simulink model "CPM"  (R2021a)
settings: Solver=VariableStepAuto  StartTime=0.0  StopTime=10.0  RelTol=1e-3
undefined symbols (not defined in the file or in its folder): robot
libraries: robotmaniplib x11, robotcorelib x2, dspinverses x1
settings Model: Creator=ajosh  LastModifiedBy=mluser
settings SolverCC: AlgebraicLoopSolver=TrustRegion
settings OptimizationCC: BlockReduction=off  DefaultParameterBehavior=Inlined  BufferReuse=off
settings DebuggingCC: SFMachineParentedDataDiag=warning

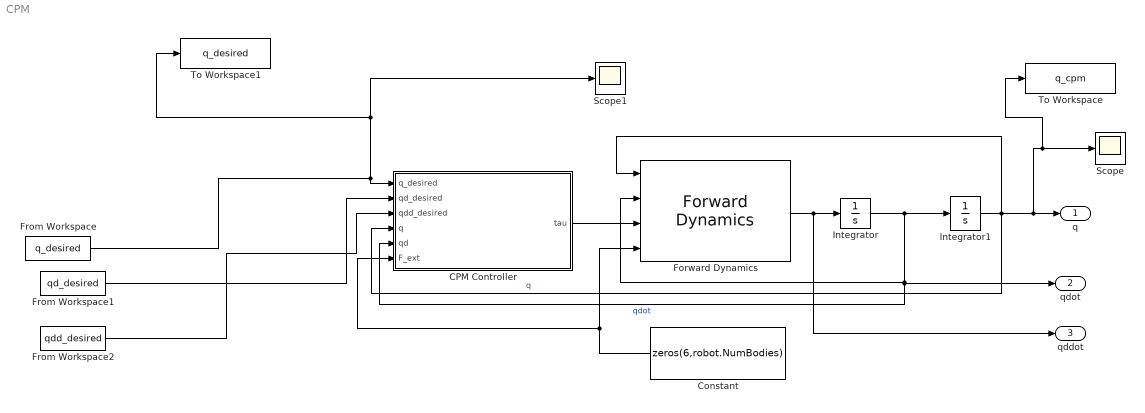
== system CPM ==
  "CPM Controller " : Subsystem
  Constant : Constant  Value=zeros(6,robot.NumBodies)
  Forward Dynamics : robotmaniplib/Forward Dynamics  RigidBodyTree=robot  SimulateUsing=Interpreted execution
  From Workspace : FromWorkspace  VariableName=q_desired  SampleTime=-1
  From Workspace1 : FromWorkspace  VariableName=qd_desired  SampleTime=-1
  From Workspace2 : FromWorkspace  VariableName=qdd_desired  SampleTime=-1
  Integrator : Integrator
  Integrator1 : Integrator
  Scope : Scope
  Scope1 : Scope
  To Workspace : ToWorkspace  VariableName=q_cpm  SaveFormat=Timeseries  SampleTime=-1
  To Workspace1 : ToWorkspace  VariableName=q_desired  SaveFormat=Timeseries  SampleTime=-1
  q : Outport
  qdot : Outport  Port=2
  qddot : Outport  Port=3
  wires:
  Forward Dynamics/1 -> Integrator/1, qddot/1
  Integrator/1 -> Integrator1/1, "CPM Controller "/5(qd), qdot/1, Forward Dynamics/2  "qdot"
  "CPM Controller "/1(tau) -> Forward Dynamics/3
  Integrator1/1 -> Forward Dynamics/1, To Workspace/1, Scope/1, q/1, "CPM Controller "/4(q)  "q"
  Constant/1 -> "CPM Controller "/6(F_ext), Forward Dynamics/4
  From Workspace/1 -> Scope1/1, To Workspace1/1, "CPM Controller "/1(q_desired)
  From Workspace1/1 -> "CPM Controller "/2(qd_desired)
  From Workspace2/1 -> "CPM Controller "/3(qdd_desired)

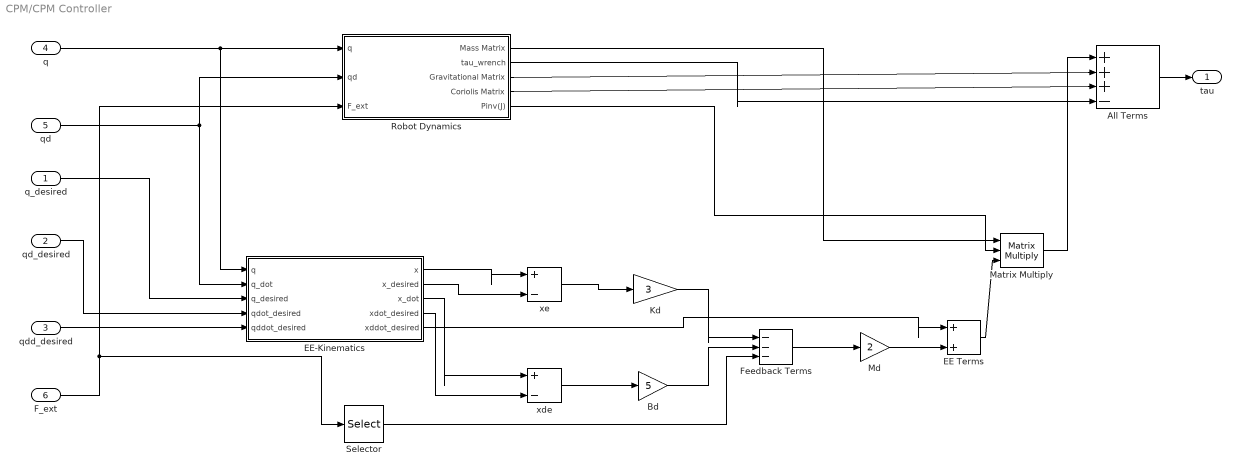
== system CPM/CPM Controller  ==
  q_desired : Inport
  qd_desired : Inport  Port=2
  qdd_desired : Inport  Port=3
  q : Inport  Port=4
  qd : Inport  Port=5
  F_ext : Inport  Port=6
  All Terms : Sum  Inputs=|+++-
  Bd : Gain  Gain=5
  EE Terms : Sum  Inputs=|++
  EE-Kinematics : Subsystem
  Feedback Terms : Sum  Inputs=|---
  Kd : Gain  Gain=3
  Matrix Multiply : Product  Inputs=3  Multiplication=Matrix(*)
  Md : Gain  Gain=2
  Robot Dynamics : Subsystem
  Selector : Selector  NumberOfDimensions=2  InputPortWidth=3  IndexOptions=Index vector (dialog),Index vector (dialog)  Indices=[1 2 3 4 5 6],2  OutputSizes=1,1
  xde : Sum  Inputs=|+-
  xe : Sum  Inputs=|+-
  tau : Outport
  wires:
  qd/1 -> EE-Kinematics/2(q_dot), Robot Dynamics/2(qd)
  xe/1 -> Kd/1
  xde/1 -> Bd/1
  Kd/1 -> Feedback Terms/1
  Bd/1 -> Feedback Terms/2
  q_desired/1 -> EE-Kinematics/3(q_desired)
  qd_desired/1 -> EE-Kinematics/4(qdot_desired)
  qdd_desired/1 -> EE-Kinematics/5(qddot_desired)
  q/1 -> EE-Kinematics/1(q), Robot Dynamics/1(q)
  EE-Kinematics/1(x) -> xe/1
  EE-Kinematics/2(x_desired) -> xe/2
  EE-Kinematics/3(x_dot) -> xde/1
  EE-Kinematics/4(xdot_desired) -> xde/2
  F_ext/1 -> Selector/1, Robot Dynamics/3(F_ext)
  Feedback Terms/1 -> Md/1
  Md/1 -> EE Terms/2
  EE-Kinematics/5(xddot_desired) -> EE Terms/1
  Robot Dynamics/1(Mass Matrix) -> Matrix Multiply/1
  Robot Dynamics/5(Pinv(J)) -> Matrix Multiply/2
  EE Terms/1 -> Matrix Multiply/3
  Matrix Multiply/1 -> All Terms/1
  Robot Dynamics/3(Gravitational Matrix) -> All Terms/2
  Robot Dynamics/2("tau_wrench ") -> All Terms/4
  All Terms/1 -> tau/1
  Robot Dynamics/4(Coriolis Matrix) -> All Terms/3
  Selector/1 -> Feedback Terms/3

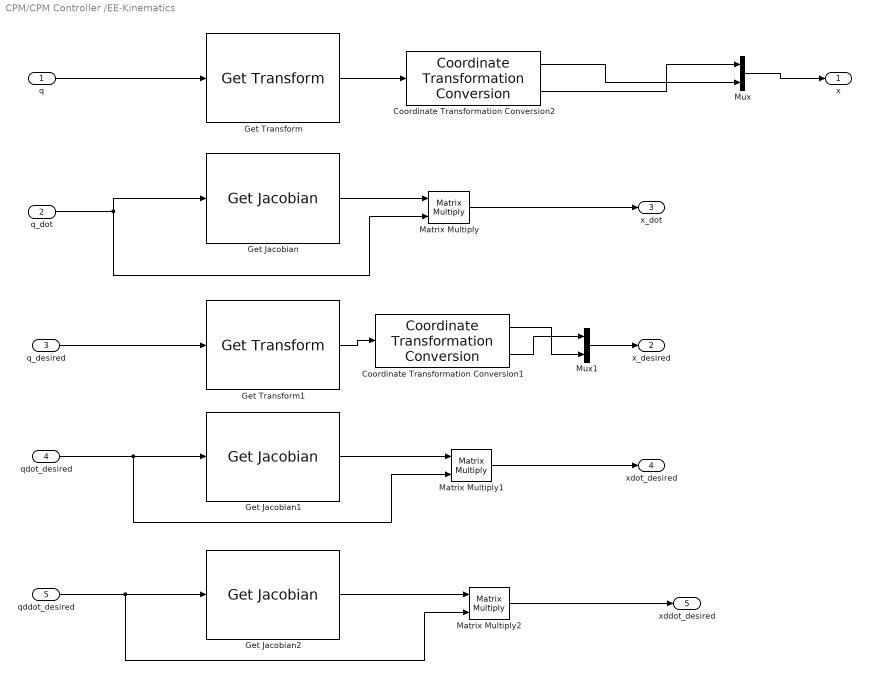
== system CPM/CPM Controller /EE-Kinematics ==
  q : Inport
  q_dot : Inport  Port=2
  q_desired : Inport  Port=3
  qdot_desired : Inport  Port=4
  qddot_desired : Inport  Port=5
  Coordinate Transformation Conversion1 : robotcorelib/Coordinate Transformation Conversion  InputRepresentation=Homogeneous Transformation  InputEulerSequence=ZYX  ShowTrVecInputPort=on  OutputRepresentation=Euler Angles  OutputEulerSequence=XYZ  ShowTrVecOutputPort=on  SimulateUsing=Interpreted execution
      settings: SourceProductBaseCode=NV,RO,RR,UV
  Coordinate Transformation Conversion2 : robotcorelib/Coordinate Transformation Conversion  InputRepresentation=Homogeneous Transformation  InputEulerSequence=ZYX  ShowTrVecInputPort=on  OutputRepresentation=Euler Angles  OutputEulerSequence=XYZ  ShowTrVecOutputPort=on  SimulateUsing=Interpreted execution
      settings: SourceProductBaseCode=NV,RO,RR,UV
  Get Jacobian : robotmaniplib/Get Jacobian  RigidBodyTree=robot  EndEffector=handle  SimulateUsing=Interpreted execution
      settings: SourceProductBaseCode=RO
  Get Jacobian1 : robotmaniplib/Get Jacobian  RigidBodyTree=robot  EndEffector=handle  SimulateUsing=Interpreted execution
      settings: SourceProductBaseCode=RO
  Get Jacobian2 : robotmaniplib/Get Jacobian  RigidBodyTree=robot  EndEffector=handle  SimulateUsing=Interpreted execution
      settings: SourceProductBaseCode=RO
  Get Transform : robotmaniplib/Get Transform  RigidBodyTree=robot  SourceBody=base_link  TargetBody=base_link  SimulateUsing=Interpreted execution
  Get Transform1 : robotmaniplib/Get Transform  RigidBodyTree=robot  SourceBody=base_link  TargetBody=base_link  SimulateUsing=Interpreted execution
  Matrix Multiply : Product  Multiplication=Matrix(*)
  Matrix Multiply1 : Product  Multiplication=Matrix(*)
  Matrix Multiply2 : Product  Multiplication=Matrix(*)
  Mux : Mux  Inputs=2
  Mux1 : Mux  Inputs=2
  x : Outport
  x_desired : Outport  Port=2
  x_dot : Outport  Port=3
  xdot_desired : Outport  Port=4
  xddot_desired : Outport  Port=5
  wires:
  q/1 -> Get Transform/1
  Get Transform/1 -> Coordinate Transformation Conversion2/1
  q_dot/1 -> Matrix Multiply/2, Get Jacobian/1
  Get Jacobian/1 -> Matrix Multiply/1
  q_desired/1 -> Get Transform1/1
  Get Transform1/1 -> Coordinate Transformation Conversion1/1
  Get Jacobian1/1 -> Matrix Multiply1/1
  qdot_desired/1 -> Matrix Multiply1/2, Get Jacobian1/1
  Get Jacobian2/1 -> Matrix Multiply2/1
  qddot_desired/1 -> Matrix Multiply2/2, Get Jacobian2/1
  Matrix Multiply2/1 -> xddot_desired/1
  Matrix Multiply1/1 -> xdot_desired/1
  Matrix Multiply/1 -> x_dot/1
  Coordinate Transformation Conversion2/2 -> Mux/1
  Coordinate Transformation Conversion2/1 -> Mux/2
  Mux/1 -> x/1
  Coordinate Transformation Conversion1/2 -> Mux1/1
  Coordinate Transformation Conversion1/1 -> Mux1/2
  Mux1/1 -> x_desired/1

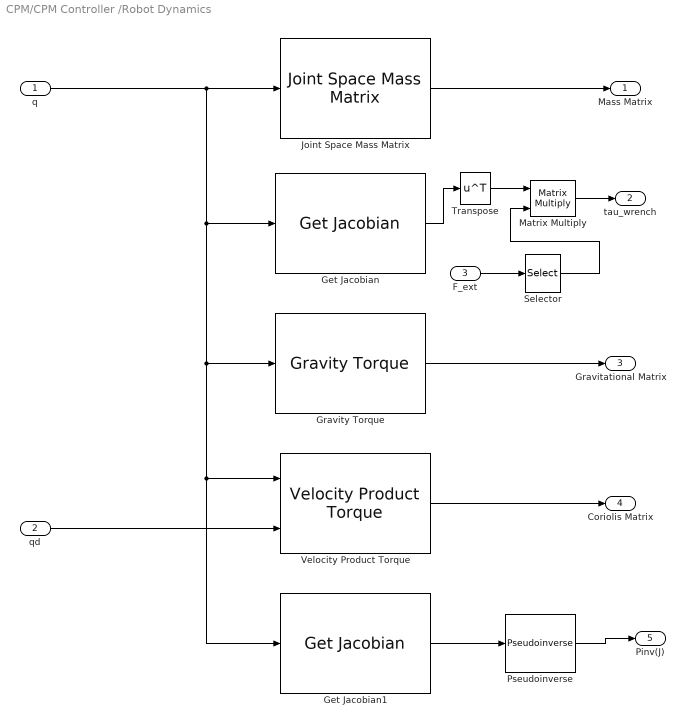
== system CPM/CPM Controller /Robot Dynamics ==
  q : Inport
  qd : Inport  Port=2
  F_ext : Inport  Port=3
  Get Jacobian : robotmaniplib/Get Jacobian  RigidBodyTree=robot  EndEffector=handle  SimulateUsing=Interpreted execution
      settings: SourceProductBaseCode=RO
  Get Jacobian1 : robotmaniplib/Get Jacobian  RigidBodyTree=robot  EndEffector=handle  SimulateUsing=Interpreted execution
      settings: SourceProductBaseCode=RO
  Gravity Torque : robotmaniplib/Gravity Torque  RigidBodyTree=robot  SimulateUsing=Interpreted execution
  Joint Space Mass Matrix : robotmaniplib/Joint Space Mass Matrix  RigidBodyTree=robot  SimulateUsing=Interpreted execution
  Matrix Multiply : Product  Multiplication=Matrix(*)
  Pseudoinverse : dspinverses/Pseudoinverse  wanterr=off  SimulateUsing=Interpreted execution
      settings: SourceProductBaseCode=DS
  Selector : Selector  NumberOfDimensions=2  InputPortWidth=3  IndexOptions=Index vector (dialog),Index vector (dialog)  Indices=[1 2 3 4 5 6],2  OutputSizes=1,1
  Transpose : Math  Operator=transpose  SaturateOnIntegerOverflow=on
  Velocity Product Torque : robotmaniplib/Velocity Product Torque  RigidBodyTree=robot  SimulateUsing=Interpreted execution
      settings: SourceProductBaseCode=RO
  Mass Matrix : Outport
  "tau_wrench " : Outport  Port=2
  Gravitational Matrix : Outport  Port=3
  Coriolis Matrix : Outport  Port=4
  Pinv(J) : Outport  Port=5
  wires:
  q/1 -> Joint Space Mass Matrix/1, Get Jacobian1/1, Velocity Product Torque/1, Gravity Torque/1, Get Jacobian/1
  Joint Space Mass Matrix/1 -> Mass Matrix/1
  Gravity Torque/1 -> Gravitational Matrix/1
  Get Jacobian/1 -> Transpose/1
  Transpose/1 -> Matrix Multiply/1
  F_ext/1 -> Selector/1
  Matrix Multiply/1 -> "tau_wrench "/1
  qd/1 -> Velocity Product Torque/2
  Velocity Product Torque/1 -> Coriolis Matrix/1
  Get Jacobian1/1 -> Pseudoinverse/1
  Pseudoinverse/1 -> Pinv(J)/1
  Selector/1 -> Matrix Multiply/2
